simulink model "Simulink_filtros"  (R2023a)
settings: Solver=VariableStepAuto  StartTime=0.0  StopTime=4/Frequency4  RelTol=1e-3
undefined symbols (not defined in the file): C, C1, C2, C3, Frequency, Frequency2, Frequency3, Frequency4, L, L1, R, R1, R2, R3, R4, Rload
libraries: spsSeriesRLCBranchLib x12, spsFourierLib x8, spsVoltageMeasurementLib x8, spsACVoltageSourceLib x4, spsGroundLib x4, sps_lib x1
settings Model: Creator=Juan Esteban  LastModifiedBy=Juan Esteban

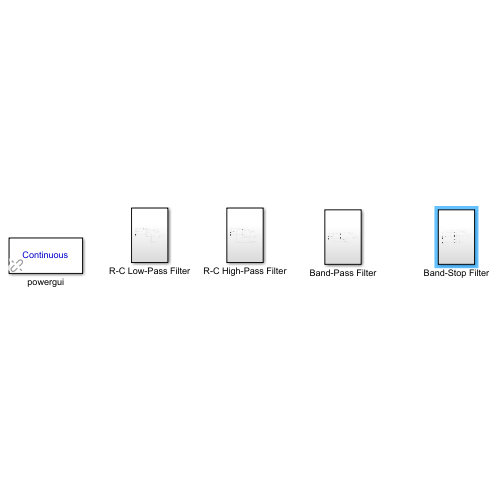
[thumbnail: Simulink's stored preview of the top-level diagram]
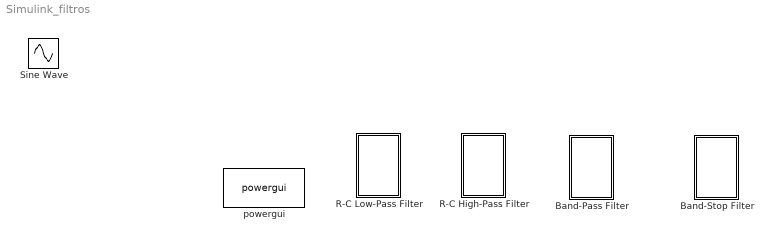
== system Simulink_filtros ==
  Band-Pass Filter : Subsystem
  "Band-Stop Filter " : Subsystem
  R-C High-Pass Filter : Subsystem
  R-C Low-Pass Filter : Subsystem
  powergui : sps_lib/powergui  Priority=1  SimulationMode=Continuous  SampleTime=50e-6  frequency=60  Iterations=50  frequencyindice=1000  Pbase=100e6  ErrMax=1e-4  UnitsV=kV  UnitsW=MW  buscounter=0  FunctionMessages=off  echomessages=off  EnableUseOfTLC=off  CurrentSourceSwitches=off  DisableSnubberDevices=off  DisableRonSwitches=off  DisableVfSwitches=off  DisplayEquations=off  AutomaticDiscreteSolvers=off  SolverType=Tustin/Backward Euler (TBE)  Interpol=off  ExternalGateDelay=off  methode=off  Ts=100  x0status=blocks  SPID=on  SwTol=0  HookPort=off  NonlinearTolerance=1e-4  nMaxIteration=100  ContinueOnMaxIteration=off  RestoreLinks=warning  ResistiveCurrentMeasurement=off  Frange=[0:2:500]  Ylog=off  Xlog=on  ShowGrid=off  save=off  variable=ZData  structure=0  ZoomFFT=off  StartTime=0.0  cycles=1  DisplayStyle=1  fundamental=60  FreqAxis=off  MaxFrequency=1000  frequencyindicesteady=1  RmsSteady=1  display=off
  Sine Wave : Sin  IOType=siggen  SampleTime=0

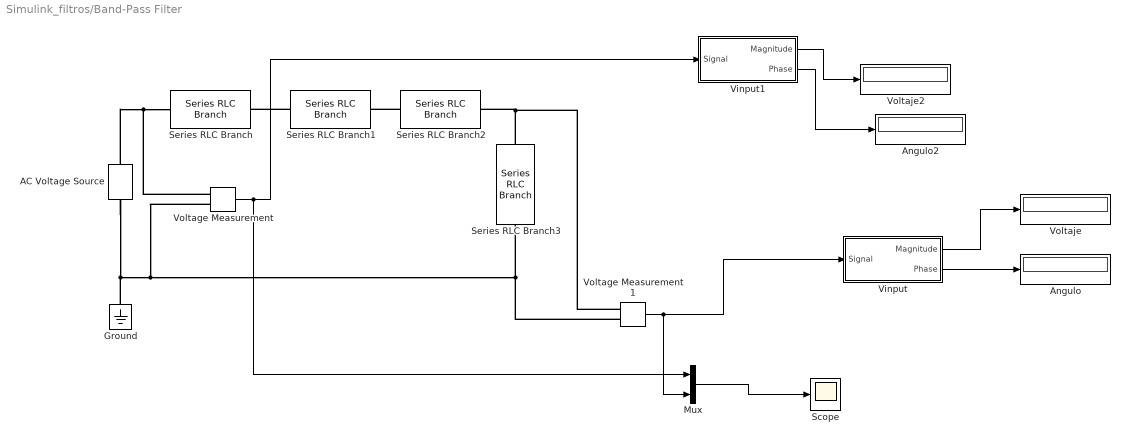
== system Simulink_filtros/Band-Pass Filter ==
  AC Voltage Source : spsACVoltageSourceLib/AC Voltage Source  Amplitude=5  Phase=0  Frequency=Frequency3  SampleTime=0  Measurements=None  BusType=swing  Pref=10e3  Qref=0  Qmin=-inf  Qmax=+inf
  Angulo : Display
  Angulo2 : Display
  Ground : spsGroundLib/Ground  LConnTagsString=a
  Mux : Mux  Inputs=2
  Scope : Scope
  Series RLC Branch : spsSeriesRLCBranchLib/Series RLC Branch  LConnTagsString=__new0  RConnTagsString=__new0  BranchType=R  Resistance=R2  Inductance=1e-3  SetiL0=off  InitialCurrent=0  Capacitance=1e-6  Setx0=off  InitialVoltage=0  Measurements=None
  Series RLC Branch1 : spsSeriesRLCBranchLib/Series RLC Branch  LConnTagsString=__new0  RConnTagsString=__new0  BranchType=L  Resistance=1  Inductance=L  SetiL0=off  InitialCurrent=0  Capacitance=1e-6  Setx0=off  InitialVoltage=0  Measurements=None
  Series RLC Branch2 : spsSeriesRLCBranchLib/Series RLC Branch  LConnTagsString=__new0  RConnTagsString=__new0  BranchType=C  Resistance=1  Inductance=1e-3  SetiL0=off  InitialCurrent=0  Capacitance=C2  Setx0=off  InitialVoltage=0  Measurements=None
  Series RLC Branch3 : spsSeriesRLCBranchLib/Series RLC Branch  LConnTagsString=__new0  RConnTagsString=__new0  BranchType=R  Resistance=Rload  Inductance=1e-3  SetiL0=off  InitialCurrent=0  Capacitance=1e-6  Setx0=off  InitialVoltage=0  Measurements=Branch voltage
  Vinput : Subsystem
  Vinput1 : Subsystem
  Voltage Measurement : spsVoltageMeasurementLib/Voltage Measurement  PhasorSimulation=off  OutputType=Complex  PSBequivalent=0
  Voltage Measurement1 : spsVoltageMeasurementLib/Voltage Measurement  PhasorSimulation=off  OutputType=Complex  PSBequivalent=0
  Voltaje : Display
  Voltaje2 : Display
  wires:
  Vinput/1(Magnitude) -> Voltaje/1
  Vinput1/1(Magnitude) -> Voltaje2/1
  Vinput/2(Phase) -> Angulo/1
  Voltage Measurement1/1 -> Mux/2, Vinput/1(Signal)
  Vinput1/2(Phase) -> Angulo2/1
  Voltage Measurement/1 -> Mux/1, Vinput1/1(Signal)
  Mux/1 -> Scope/1
  connections:
  AC Voltage Source/RConn1 -- Voltage Measurement/LConn1 -- Series RLC Branch/LConn1
  AC Voltage Source/LConn1 -- Ground/LConn1 -- Voltage Measurement/LConn2 -- Voltage Measurement1/LConn2 -- Series RLC Branch3/RConn1
  Series RLC Branch1/LConn1 -- Series RLC Branch/RConn1
  Series RLC Branch2/LConn1 -- Series RLC Branch1/RConn1
  Series RLC Branch3/LConn1 -- Voltage Measurement1/LConn1 -- Series RLC Branch2/RConn1

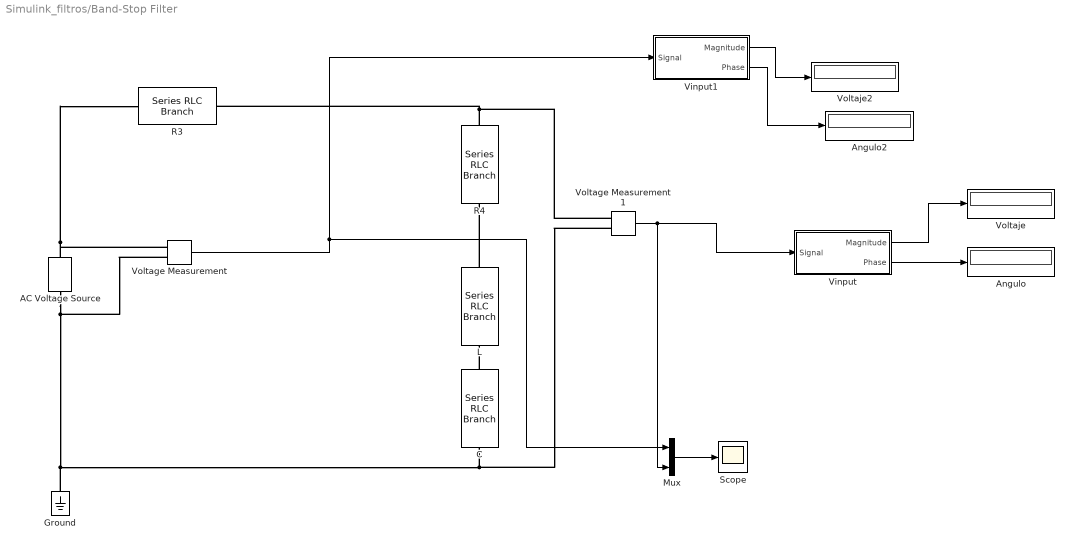
== system Simulink_filtros/Band-Stop Filter  ==
  AC Voltage Source : spsACVoltageSourceLib/AC Voltage Source  Amplitude=5  Phase=0  Frequency=Frequency4  SampleTime=0  Measurements=None  BusType=swing  Pref=10e3  Qref=0  Qmin=-inf  Qmax=+inf
  Angulo : Display
  Angulo2 : Display
  C : spsSeriesRLCBranchLib/Series RLC Branch  LConnTagsString=__new0  RConnTagsString=__new0  BranchType=C  Resistance=Rload  Inductance=1e-3  SetiL0=off  InitialCurrent=0  Capacitance=C3  Setx0=off  InitialVoltage=0  Measurements=Branch voltage
  Ground : spsGroundLib/Ground  LConnTagsString=a
  L : spsSeriesRLCBranchLib/Series RLC Branch  LConnTagsString=__new0  RConnTagsString=__new0  BranchType=L  Resistance=1  Inductance=L1  SetiL0=off  InitialCurrent=0  Capacitance=C2  Setx0=off  InitialVoltage=0  Measurements=None
  Mux : Mux  Inputs=2
  R3 : spsSeriesRLCBranchLib/Series RLC Branch  LConnTagsString=__new0  RConnTagsString=__new0  BranchType=R  Resistance=R3  Inductance=1e-3  SetiL0=off  InitialCurrent=0  Capacitance=1e-6  Setx0=off  InitialVoltage=0  Measurements=None
  R4 : spsSeriesRLCBranchLib/Series RLC Branch  LConnTagsString=__new0  RConnTagsString=__new0  BranchType=R  Resistance=R4  Inductance=L  SetiL0=off  InitialCurrent=0  Capacitance=1e-6  Setx0=off  InitialVoltage=0  Measurements=Branch voltage
  Scope : Scope
  Vinput : Subsystem
  Vinput1 : Subsystem
  Voltage Measurement : spsVoltageMeasurementLib/Voltage Measurement  PhasorSimulation=off  OutputType=Complex  PSBequivalent=0
  Voltage Measurement1 : spsVoltageMeasurementLib/Voltage Measurement  PhasorSimulation=off  OutputType=Complex  PSBequivalent=0
  Voltaje : Display
  Voltaje2 : Display
  wires:
  Vinput/1(Magnitude) -> Voltaje/1
  Vinput1/1(Magnitude) -> Voltaje2/1
  Vinput/2(Phase) -> Angulo/1
  Vinput1/2(Phase) -> Angulo2/1
  Voltage Measurement/1 -> Mux/1, Vinput1/1(Signal)
  Voltage Measurement1/1 -> Mux/2, Vinput/1(Signal)
  Mux/1 -> Scope/1
  connections:
  AC Voltage Source/RConn1 -- R3/LConn1 -- Voltage Measurement/LConn1
  R4/LConn1 -- Voltage Measurement1/LConn1 -- R3/RConn1
  L/LConn1 -- R4/RConn1
  C/LConn1 -- L/RConn1
  Voltage Measurement1/LConn2 -- Voltage Measurement/LConn2 -- AC Voltage Source/LConn1 -- Ground/LConn1 -- C/RConn1

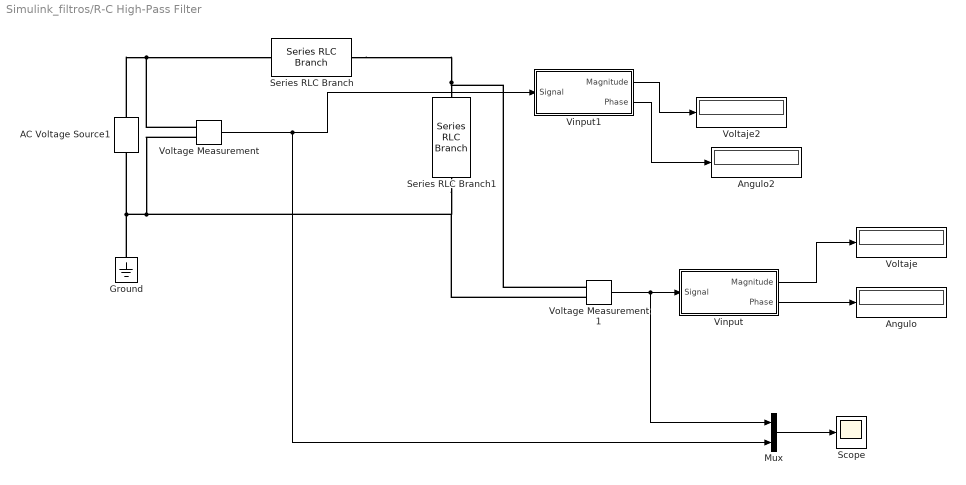
== system Simulink_filtros/R-C High-Pass Filter ==
  AC Voltage Source1 : spsACVoltageSourceLib/AC Voltage Source  Amplitude=5  Phase=0  Frequency=Frequency2  SampleTime=0  Measurements=None  BusType=swing  Pref=10e3  Qref=0  Qmin=-inf  Qmax=+inf
  Angulo : Display
  Angulo2 : Display
  Ground : spsGroundLib/Ground  LConnTagsString=a
  Mux : Mux  Inputs=2
  Scope : Scope
  Series RLC Branch : spsSeriesRLCBranchLib/Series RLC Branch  LConnTagsString=__new0  RConnTagsString=__new0  BranchType=C  Resistance=R  Inductance=1e-3  SetiL0=off  InitialCurrent=0  Capacitance=C1  Setx0=off  InitialVoltage=0  Measurements=None
  Series RLC Branch1 : spsSeriesRLCBranchLib/Series RLC Branch  LConnTagsString=__new0  RConnTagsString=__new0  BranchType=R  Resistance=R1  Inductance=1e-3  SetiL0=off  InitialCurrent=0  Capacitance=C  Setx0=off  InitialVoltage=0  Measurements=Branch voltage
  Vinput : Subsystem
  Vinput1 : Subsystem
  Voltage Measurement : spsVoltageMeasurementLib/Voltage Measurement  PhasorSimulation=off  OutputType=Complex  PSBequivalent=0
  Voltage Measurement1 : spsVoltageMeasurementLib/Voltage Measurement  PhasorSimulation=off  OutputType=Complex  PSBequivalent=0
  Voltaje : Display
  Voltaje2 : Display
  wires:
  Vinput/2(Phase) -> Angulo/1
  Vinput1/2(Phase) -> Angulo2/1
  Vinput/1(Magnitude) -> Voltaje/1
  Vinput1/1(Magnitude) -> Voltaje2/1
  Voltage Measurement/1 -> Mux/2, Vinput1/1(Signal)
  Mux/1 -> Scope/1
  Voltage Measurement1/1 -> Mux/1, Vinput/1(Signal)
  connections:
  Voltage Measurement/LConn2 -- Series RLC Branch1/RConn1 -- Voltage Measurement1/LConn2 -- Ground/LConn1 -- AC Voltage Source1/LConn1
  Voltage Measurement/LConn1 -- AC Voltage Source1/RConn1 -- Series RLC Branch/LConn1
  Series RLC Branch/RConn1 -- Voltage Measurement1/LConn1 -- Series RLC Branch1/LConn1

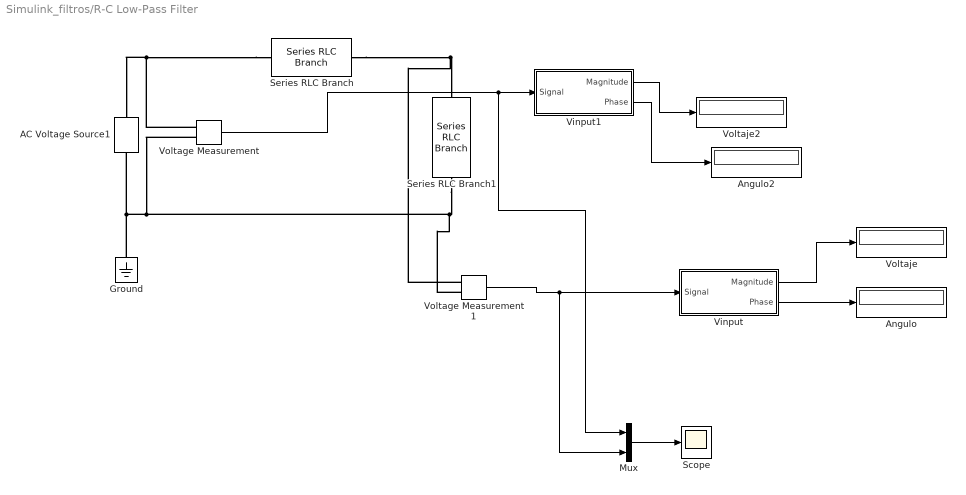
== system Simulink_filtros/R-C Low-Pass Filter ==
  AC Voltage Source1 : spsACVoltageSourceLib/AC Voltage Source  Amplitude=5  Phase=0  Frequency=Frequency  SampleTime=0  Measurements=None  BusType=swing  Pref=10e3  Qref=0  Qmin=-inf  Qmax=+inf
  Angulo : Display
  Angulo2 : Display
  Ground : spsGroundLib/Ground  LConnTagsString=a
  Mux : Mux  Inputs=2
  Scope : Scope
  Series RLC Branch : spsSeriesRLCBranchLib/Series RLC Branch  LConnTagsString=__new0  RConnTagsString=__new0  BranchType=R  Resistance=R  Inductance=1e-3  SetiL0=off  InitialCurrent=0  Capacitance=1e-6  Setx0=off  InitialVoltage=0  Measurements=None
  Series RLC Branch1 : spsSeriesRLCBranchLib/Series RLC Branch  LConnTagsString=__new0  RConnTagsString=__new0  BranchType=C  Resistance=1  Inductance=1e-3  SetiL0=off  InitialCurrent=0  Capacitance=C  Setx0=off  InitialVoltage=0  Measurements=Branch voltage
  Vinput : Subsystem
  Vinput1 : Subsystem
  Voltage Measurement : spsVoltageMeasurementLib/Voltage Measurement  PhasorSimulation=off  OutputType=Complex  PSBequivalent=0
  Voltage Measurement1 : spsVoltageMeasurementLib/Voltage Measurement  PhasorSimulation=off  OutputType=Complex  PSBequivalent=0
  Voltaje : Display
  Voltaje2 : Display
  wires:
  Vinput/2(Phase) -> Angulo/1
  Vinput1/2(Phase) -> Angulo2/1
  Vinput/1(Magnitude) -> Voltaje/1
  Vinput1/1(Magnitude) -> Voltaje2/1
  Voltage Measurement/1 -> Mux/1, Vinput1/1(Signal)
  Mux/1 -> Scope/1
  Voltage Measurement1/1 -> Mux/2, Vinput/1(Signal)
  connections:
  AC Voltage Source1/LConn1 -- Ground/LConn1 -- Voltage Measurement1/LConn2 -- Series RLC Branch1/RConn1 -- Voltage Measurement/LConn2
  Series RLC Branch/RConn1 -- Voltage Measurement1/LConn1 -- Series RLC Branch1/LConn1
  Series RLC Branch/LConn1 -- AC Voltage Source1/RConn1 -- Voltage Measurement/LConn1

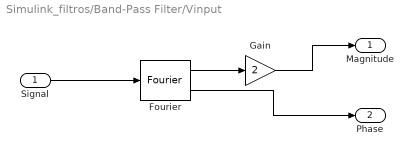
== system Simulink_filtros/Band-Pass Filter/Vinput ==
  Signal : Inport
  Fourier : spsFourierLib/Fourier  Freq=Frequency3  n=1  InInit=[0, 0]  Ts=0
  Gain : Gain  Gain=2
  Magnitude : Outport
  Phase : Outport  Port=2
  wires:
  Fourier/1 -> Gain/1
  Fourier/2 -> Phase/1
  Gain/1 -> Magnitude/1
  Signal/1 -> Fourier/1

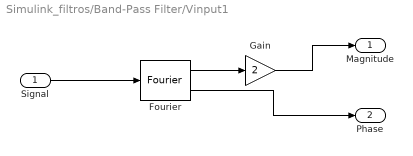
== system Simulink_filtros/Band-Pass Filter/Vinput1 ==
  Signal : Inport
  Fourier : spsFourierLib/Fourier  Freq=Frequency3  n=1  InInit=[0, 0]  Ts=0
  Gain : Gain  Gain=2
  Magnitude : Outport
  Phase : Outport  Port=2
  wires:
  Fourier/1 -> Gain/1
  Fourier/2 -> Phase/1
  Gain/1 -> Magnitude/1
  Signal/1 -> Fourier/1

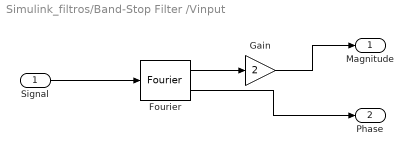
== system Simulink_filtros/Band-Stop Filter /Vinput ==
  Signal : Inport
  Fourier : spsFourierLib/Fourier  Freq=Frequency4  n=1  InInit=[0, 0]  Ts=0
  Gain : Gain  Gain=2
  Magnitude : Outport
  Phase : Outport  Port=2
  wires:
  Fourier/1 -> Gain/1
  Fourier/2 -> Phase/1
  Gain/1 -> Magnitude/1
  Signal/1 -> Fourier/1

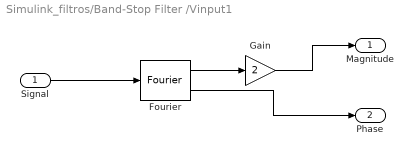
== system Simulink_filtros/Band-Stop Filter /Vinput1 ==
  Signal : Inport
  Fourier : spsFourierLib/Fourier  Freq=Frequency4  n=1  InInit=[0, 0]  Ts=0
  Gain : Gain  Gain=2
  Magnitude : Outport
  Phase : Outport  Port=2
  wires:
  Fourier/1 -> Gain/1
  Fourier/2 -> Phase/1
  Gain/1 -> Magnitude/1
  Signal/1 -> Fourier/1

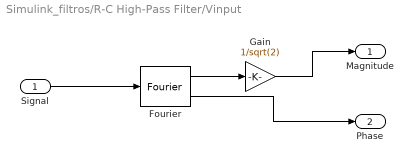
== system Simulink_filtros/R-C High-Pass Filter/Vinput ==
  Signal : Inport
  Fourier : spsFourierLib/Fourier  Freq=Frequency2  n=1  InInit=[0, 0]  Ts=0
  Gain : Gain  Gain=1/sqrt(2)
  Magnitude : Outport
  Phase : Outport  Port=2
  wires:
  Fourier/1 -> Gain/1
  Fourier/2 -> Phase/1
  Gain/1 -> Magnitude/1
  Signal/1 -> Fourier/1

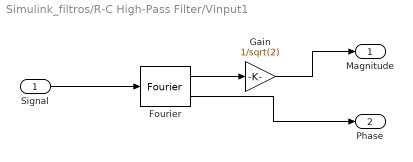
== system Simulink_filtros/R-C High-Pass Filter/Vinput1 ==
  Signal : Inport
  Fourier : spsFourierLib/Fourier  Freq=Frequency2  n=1  InInit=[0, 0]  Ts=0
  Gain : Gain  Gain=1/sqrt(2)
  Magnitude : Outport
  Phase : Outport  Port=2
  wires:
  Fourier/1 -> Gain/1
  Fourier/2 -> Phase/1
  Gain/1 -> Magnitude/1
  Signal/1 -> Fourier/1

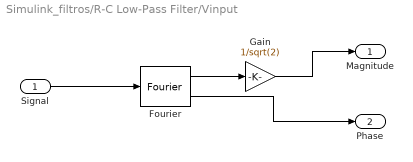
== system Simulink_filtros/R-C Low-Pass Filter/Vinput ==
  Signal : Inport
  Fourier : spsFourierLib/Fourier  Freq=Frequency  n=1  InInit=[0, 0]  Ts=0
  Gain : Gain  Gain=1/sqrt(2)
  Magnitude : Outport
  Phase : Outport  Port=2
  wires:
  Fourier/1 -> Gain/1
  Fourier/2 -> Phase/1
  Gain/1 -> Magnitude/1
  Signal/1 -> Fourier/1

== system Simulink_filtros/R-C Low-Pass Filter/Vinput1 ==
  Signal : Inport
  Fourier : spsFourierLib/Fourier  Freq=Frequency  n=1  InInit=[0, 0]  Ts=0
  Gain : Gain  Gain=1/sqrt(2)
  Magnitude : Outport
  Phase : Outport  Port=2
  wires:
  Fourier/1 -> Gain/1
  Fourier/2 -> Phase/1
  Gain/1 -> Magnitude/1
  Signal/1 -> Fourier/1
